simulink model "UE03_b_2"  (R2022b)
settings: Solver=VariableStepAuto  StartTime=0.0  StopTime=10.0  RelTol=1e-3
settings Model: Creator=basti  LastModifiedBy=basti

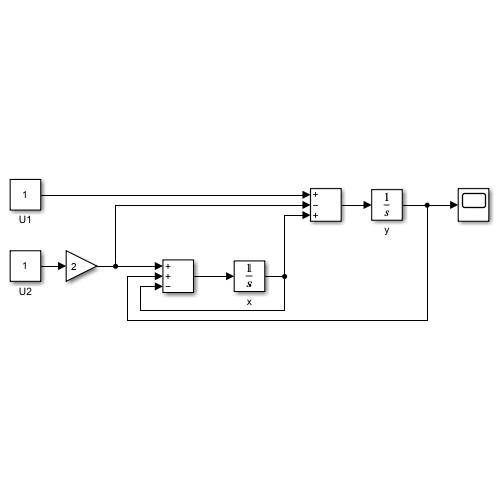
[thumbnail: Simulink's stored preview of the top-level diagram]
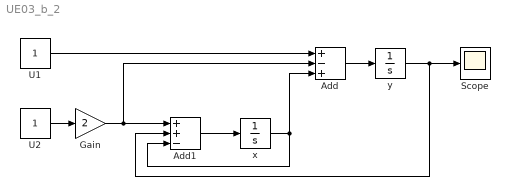
== system UE03_b_2 ==
  Add : Sum  Inputs=+-+
  Add1 : Sum  Inputs=++-
  Gain : Gain  Gain=2
  Scope : Scope
  U1 : Constant
  U2 : Constant
  x : Integrator
  y : Integrator
  wires:
  Gain/1 -> Add/2, Add1/1
  U2/1 -> Gain/1
  U1/1 -> Add/1
  Add1/1 -> x/1
  x/1 -> Add/3, Add1/3
  Add/1 -> y/1
  y/1 -> Add1/2, Scope/1
